simulink model "Model_6DOF_B3"  (R2020b)
settings: Solver=FixedStepAuto  StartTime=0.0  StopTime=120  FixedStep=0.05  RelTol=1e-3
values from neighbouring files (symbols this model uses):
  Ba_0 = [0 0 0 0 0 0]    [ctrl_mode_param.m]
  Bb = 4418825.3321    [load_data.m]
  Bv_0 = [tgt_speed 0 0 0 0 0]    [ctrl_mode_param.m]
  Bx_0 = [0 0 tgt_depth 0 0 0]    [ctrl_mode_param.m]
  Ixx = 5.23e7    (= 52300000)    [load_data.m]
  Ixy = 0    [load_data.m]
  Ixz = 0    [load_data.m]
  Iyy = 1.375e9    (= 1375000000)    [load_data.m]
  Iyz = 0    [load_data.m]
  Izz = 1.367e9    (= 1367000000)    [load_data.m]
  Mb = 4418825.3321    [load_data.m]
  Xb = 0    [load_data.m]
  Xg = 0    [load_data.m]
  Yb = 0    [load_data.m]
  Yg = 0    [load_data.m]
  Zb = 0.4406    [load_data.m]
  Zg = 0    [load_data.m]
undefined symbols (not defined in the file or in its folder): dA_BP1, dA_BP2, dA_Hull, dA_PH, dA_Sail, dA_SProot, dA_X1a, dA_X1b, dA_X2a, dA_X2b, dA_X3a, dA_X3b, dA_X4a, dA_X4b, its, n_BP1, n_BP2, n_Hull, n_PH, n_Sail, n_SProot, n_X1a, n_X1b, n_X2a, n_X2b, n_X3a, n_X3b, n_X4a, n_X4b, nt_BP1, nt_BP2, nt_Hull, nt_PH, nt_Sail, nt_SProot, nt_X1a, nt_X1b, nt_X2a, nt_X2b, nt_X3a, nt_X3b, nt_X4a, nt_X4b, Usp, vt1_BP1, vt1_BP2, vt1_Hull, vt1_PH, vt1_Sail, vt1_SProot, vt1_X1a, vt1_X1b, vt1_X2a, vt1_X2b, vt1_X3a, vt1_X3b, vt1_X4a, vt1_X4b, vt2_BP1, vt2_BP2 ... (+27)
libraries: simulink x5
(part 3 of 15)

== system Model_6DOF_B3/HDM 6DOF V1/Z 6d org ==
  Bx : Inport
  Bv : Inport  Port=2
  Ba : Inport  Port=3
  Alpha : Inport  Port=4
  Umag : Inport  Port=5
  dX : Inport  Port=6
  UeX : Inport  Port=7
  dLCG : Inport  Port=8
  dmass : Inport  Port=9
  Zvm : Inport  Port=10
  Fz : MATLAB Function  TreatAsAtomicUnit=on
  Product1 : Product
  Product3 : Product
  Saturation1 : Saturate  UpperLimit=0.04  LowerLimit=-0.04
  Saturation2 : Saturate  UpperLimit=0.0015  LowerLimit=-0.0015
  Saturation3 : Saturate  UpperLimit=0.02  LowerLimit=-0.02
  Selector1 : Selector  InputPortWidth=6  IndexOptions=Index vector (dialog)  Indices=3  OutputSizes=1
  Selector2 : Selector  InputPortWidth=6  IndexOptions=Index vector (dialog)  Indices=5  OutputSizes=1
  Selector3 : Selector  InputPortWidth=6  IndexOptions=Index vector (dialog)  Indices=3  OutputSizes=1
  Selector4 : Selector  InputPortWidth=6  IndexOptions=Index vector (dialog)  Indices=3  OutputSizes=1
  Selector7 : Selector  InputPortWidth=6  IndexOptions=Index vector (dialog)  Indices=1  OutputSizes=1
  To Workspace : ToWorkspace  VariableName=Zapp  SaveFormat=Timeseries  SampleTime=-1
  To Workspace1 : ToWorkspace  VariableName=Ztotal  SaveFormat=Timeseries  SampleTime=-1
  To Workspace2 : ToWorkspace  VariableName=Zstat  SaveFormat=Timeseries  SampleTime=-1
  To Workspace3 : ToWorkspace  VariableName=Zprop  SaveFormat=Timeseries  SampleTime=-1
  To Workspace4 : ToWorkspace  VariableName=Zhull  SaveFormat=Timeseries  SampleTime=-1
  Z'dwdt : MATLAB Function  TreatAsAtomicUnit=on
  Z'uq Prop : Lookup_n-D  BreakpointsForDimension1=|  BreakpointsForDimension2=[-7.71666 -5.14444 -3.086664 -1.543332]  Table=|  InternalRulePriority=Speed  RndMeth=Simplest  InputSameDT=on
      BreakpointsForDimension1=|
      | [-2.0E-01
      | -1.5E-01
      | -1.0E-01
      | -5.0E-02
      | 0.0E+00
      | 5.0E-02
      | 1.0E-01
      | 1.5E-01
      | 2.0E-01
      | ]
      Table=|
      | reshape([1.3913E-04
      | 1.0452E-04
      | 6.9900E-05
      | 3.5283E-05
      | 6.6700E-07
      | -3.3949E-05
      | -6.8566E-05
      | -1.0318E-04
      | -1.3780E-04
      | 2.8914E-04
      | 2.1702E-04
      | 1.4490E-04
      | 7.2785E-05
      | 6.6700E-07
      | -7.1451E-05
      | -1.4357E-04
      | -2.1569E-04
      | -2.8780E-04
      | 1.1606E-04
      | 8.7208E-05
      | 5.8361E-05
      | 2.9514E-05
      | 6.6700E-07
      | -2.8180E-05
      | -5.7027E-05
      | -8.5874E-05
      | -1.1472E-04
      | 1.1606E-04
      | 8.7208E-05
      | 5.8361E-05
      | 2.9514E-05
      | 6.6700E-07
      | -2.8180E-05
      | -5.7027E-05
      | -8.5874E-05
      | -1.1472E-04],[9,4])
      settings: InputPortMap=u0,u1
  Z'uvw : Lookup_n-D  NumberOfTableDimensions=3  BreakpointsForDimension1=|  BreakpointsForDimension2=|  BreakpointsForDimension3=|  Table=|  InternalRulePriority=Speed  RndMeth=Simplest  InputSameDT=on
      BreakpointsForDimension1=|
      | [-24
      | -16
      | -8
      | 0
      | 8
      | 16
      | 24]
      BreakpointsForDimension2=|
      | [-5.1444E+00
      | -3.0866E+00
      | -1.5433E+00
      | ]
      Table=|
      | reshape([-7.6517E-03
      | -4.8509E-03
      | -2.1091E-03
      | 3.8840E-04
      | 2.9798E-03
      | 6.0809E-03
      | 8.2821E-03
      | -7.5270E-03
      | -4.7702E-03
      | -1.9652E-03
      | 3.8840E-04
      | 2.9512E-03
      | 6.0573E-03
      | 8.1333E-03
      | -7.5193E-03
      | -4.5800E-03
      | -1.6681E-03
      | 3.8840E-04
      | 2.7791E-03
      | 5.8231E-03
      | 8.3050E-03
      | -6.2244E-03
      | -3.6100E-03
      | -9.9571E-04
      | 1.6186E-03
      | 4.2329E-03
      | 6.8473E-03
      | 9.4616E-03
      | -5.2515E-03
      | -2.9614E-03
      | -6.7142E-04
      | 1.6186E-03
      | 3.9086E-03
      | 6.1987E-03
      | 8.4887E-03
      | -4.1283E-03
      | -2.2126E-03
      | -2.9701E-04
      | 1.6186E-03
      | 3.5342E-03
      | 5.4499E-03
      | 7.3655E-03
      | -6.1999E-03
      | -3.5260E-03
      | -8.5205E-04
      | 1.8219E-03
      | 4.4958E-03
      | 7.1698E-03
      | 9.8437E-03
      | -4.9811E-03
      | -2.7134E-03
      | -4.4577E-04
      | 1.8219E-03
      | 4.0896E-03
      | 6.3572E-03
      | 8.6249E-03
      | -5.2821E-03
      | -2.9141E-03
      | -5.4610E-04
      | 1.8219E-03
      | 4.1899E-03
      | 6.5579E-03
      | 8.9259E-03
      | -6.1195E-03
      | -3.4239E-03
      | -7.2823E-04
      | 1.9674E-03
      | 4.6630E-03
      | 7.3587E-03
      | 1.0054E-02
      | -4.7022E-03
      | -2.4512E-03
      | -2.0024E-04
      | 1.9674E-03
      | 4.2184E-03
      | 6.4693E-03
      | 8.7203E-03
      | -3.4515E-03
      | -1.6452E-03
      | 1.6111E-04
      | 1.9674E-03
      | 3.7737E-03
      | 5.5800E-03
      | 7.3863E-03],[7,3,4])
      BreakpointsForDimension3=|
      | [-35.0624 -18.3724 -15.3724 -13.8724
      | ]
      settings: InputPortMap=u0,u1,u2
  ZdXi : Subsystem
  Zqq : Lookup_n-D  NumberOfTableDimensions=1  BreakpointsForDimension1=|  Table=|  InternalRulePriority=Speed  RndMeth=Simplest  InputSameDT=on
      BreakpointsForDimension1=|
      | [-0.02
      | -0.015
      | -0.012958963
      | -0.009719222
      | -0.006479482
      | -0.003239741
      | -0.00161987
      | -0.000647948
      | 0.000647948
      | 0.00161987
      | 0.003239741
      | 0.006479482
      | 0.009719222
      | 0.012958963
      | 0.015
      | 0.02
      | ]
      Table=|
      | [3.6478E-03
      | 3.8686E-03
      | 3.4313E-03
      | 4.0790E-03
      | 3.9500E-03
      | 3.6018E-03
      | 3.6796E-03
      | 3.5502E-03
      | 3.4310E-03
      | 3.4872E-03
      | 4.2239E-03
      | 4.0934E-03
      | 3.0314E-03
      | 2.5726E-03
      | 2.9188E-03
      | 2.7740E-03
      | ]
  Zuq : Lookup_n-D  NumberOfTableDimensions=1  BreakpointsForDimension1=|  Table=|  InternalRulePriority=Speed  RndMeth=Simplest  InputSameDT=on
      BreakpointsForDimension1=|
      | [-0.04
      | -0.03
      | -0.02
      | -0.01
      | -0.005
      | -0.002
      | 0.002
      | 0.005
      | 0.01
      | 0.02
      | 0.03
      | 0.04
      | ]
      Table=|
      | [-9.8908E-03
      | -9.0784E-03
      | -8.9566E-03
      | -1.0733E-02
      | -1.4141E-02
      | -2.4189E-02
      | -6.5605E-03
      | -7.1594E-03
      | -7.6366E-03
      | -7.9008E-03
      | -6.1794E-03
      | -6.1029E-03
      | ]
  Zwq : Lookup_n-D  NumberOfTableDimensions=1  BreakpointsForDimension1=|  Table=|  InternalRulePriority=Speed  RndMeth=Simplest  InputSameDT=on
      BreakpointsForDimension1=|
      | [-0.0015
      | -0.0012
      | -0.0009
      | -0.0006
      | -0.0003
      | -0.0001
      | 0.0001
      | 0.0003
      | 0.0006
      | 0.0009
      | 0.0012
      | 0.0015]
      Table=|
      | [-2.9784E-01
      | -2.6725E-01
      | -2.3292E-01
      | -2.0077E-01
      | -1.1489E-01
      | -7.6673E-03
      | -7.5516E-03
      | -1.1617E-01
      | -2.0077E-01
      | -2.9128E-01
      | -3.5974E-01
      | -4.7839E-01]
  Z : Outport
  wires:
  Selector7/1 -> Z'uvw/2, Z'uq Prop/2, Product3/2
  Selector2/1 -> Product1/1, Saturation3/1, Product3/1
  Alpha/1 -> Z'uvw/1
  Bv/1 -> Selector7/1, Selector3/1, Selector2/1, Fz/2(Bv)
  Umag/1 -> Fz/10(Umag)
  Bx/1 -> Selector4/1, Fz/1(Bx)
  Product3/1 -> Saturation1/1, Z'uq Prop/1
  UeX/1 -> Fz/11(UeX)
  Selector3/1 -> Product1/2
  Product1/1 -> Saturation2/1
  Ba/1 -> Selector1/1, Fz/3(Ba)
  dLCG/1 -> Fz/12(dLCG)
  dmass/1 -> Fz/13(dmass)
  Selector1/1 -> Z'dwdt/1(a3)
  dX/1 -> ZdXi/1(dX)
  Saturation1/1 -> Zuq/1
  Saturation2/1 -> Zwq/1
  Saturation3/1 -> Zqq/1
  Zwq/1 -> Fz/6(Zwq)
  Fz/1(FZ) -> To Workspace1/1, Z/1
  Zqq/1 -> Fz/4(Zqq)
  Zuq/1 -> Fz/5(Zuq)
  ZdXi/1(ZdX) -> Fz/14(ZdXi)
  Z'dwdt/1(Zdwdt) -> Fz/9(Zdwdt)
  Z'uq Prop/1 -> Fz/8(CZProp)
  Zvm/1 -> Fz/15(Zvm)
  Selector4/1 -> ZdXi/2(z), Z'uvw/3
  Z'uvw/1 -> Fz/7(Zuvw)
  Fz/2(FZApp) -> To Workspace/1
  Fz/5(FZhull) -> To Workspace4/1
  Fz/4(FZprop) -> To Workspace3/1
  Fz/3(FZstat) -> To Workspace2/1

== system Model_6DOF_B3/HDM B1/Effective Veloicity Calclation ==
  Bv : Inport
  uwsXi : Inport  Port=2
  uwsCG : Inport  Port=3
  Add{,1..4} (5 alike) : Sum
  Demux : Demux  Outputs=5
  Demux1 : Demux  Outputs=3
  Demux2 : Demux  Outputs=5
  Gain : Gain
  Gain1 : Gain
  Gain2 : Gain
  MATLAB Function : MATLAB Function  TreatAsAtomicUnit=on
  MATLAB Function1 : MATLAB Function  TreatAsAtomicUnit=on
  MATLAB Function2 : MATLAB Function  TreatAsAtomicUnit=on
  X_SP1 : Constant  Value=[31.924; 3.861; -3.861;]
  X_SP2 : Constant  Value=[31.924; 3.861; 3.861;]
  X_SP3 : Constant  Value=[31.924; -3.861; 3.861;]
  X_SP4 : Constant  Value=[31.924; -3.861; -3.861;]
  X_XB : Constant  Value=[-10.465; 0; 9.732;]
  aX : Scope  NumInputPorts=5
  n1 : Constant  Value=[0; 1/sqrt(2); -1/sqrt(2);]
  n2 : Constant  Value=[0; 1/sqrt(2); 1/sqrt(2);]
  n3 : Constant  Value=[0; -1/sqrt(2); 1/sqrt(2);]
  n4 : Constant  Value=[0; -1/sqrt(2); -1/sqrt(2);]
  n5 : Constant  Value=[0; 1; 0;]
  nh : Constant  Value=[-1; 0; 0;]
  urXi : Scope  NumInputPorts=5
  Alpha : Outport
  Beta : Outport  Port=2
  Umag : Outport  Port=3
  aXi : Outport  Port=4
  UeX : Outport  Port=5
  wires:
  uwsXi/1 -> Gain2/1
  Gain2/1 -> Demux/1
  Gain1/1 -> aXi/1
  Gain/1 -> Alpha/1
  uwsCG/1 -> Demux1/1
  Demux2/5 -> aX/5
  Demux2/4 -> aX/4
  Demux2/3 -> aX/3
  Demux2/2 -> aX/2
  Demux2/1 -> aX/1
  Demux1/3 -> MATLAB Function2/4(wCG)
  Demux1/2 -> MATLAB Function2/3(vCG)
  Demux1/1 -> MATLAB Function2/2(uCG)
  MATLAB Function/2(UeX) -> UeX/1
  MATLAB Function2/3(Umag) -> Umag/1
  MATLAB Function2/2(beta) -> Beta/1
  MATLAB Function2/1(alpha) -> Gain/1
  MATLAB Function1/2(urX2) -> urXi/2, Add1/1
  MATLAB Function1/3(urX3) -> urXi/3, Add2/1
  MATLAB Function1/4(urX4) -> urXi/4, Add3/1
  MATLAB Function1/5(urXB) -> urXi/5, Add4/1
  Demux/5 -> Add4/2
  Demux/4 -> Add3/2
  Demux/3 -> Add2/2
  Demux/2 -> Add1/2
  Add4/1 -> MATLAB Function/11(urXB)
  Add3/1 -> MATLAB Function/10(urX4)
  Add2/1 -> MATLAB Function/9(urX3)
  Add1/1 -> MATLAB Function/8(urX2)
  Add/1 -> MATLAB Function/7(urX1)
  Demux/1 -> Add/2
  MATLAB Function/1(aX) -> Demux2/1, Gain1/1
  MATLAB Function1/1(urX1) -> urXi/1, Add/1
  n5/1 -> MATLAB Function/6(nB)
  X_SP1/1 -> MATLAB Function1/1(rX1)
  X_SP4/1 -> MATLAB Function1/4(rX4)
  X_SP3/1 -> MATLAB Function1/3(rX3)
  X_SP2/1 -> MATLAB Function1/2(rX2)
  X_XB/1 -> MATLAB Function1/5(rXB)
  n4/1 -> MATLAB Function/5(n4)
  n3/1 -> MATLAB Function/4(n3)
  n2/1 -> MATLAB Function/3(n2)
  n1/1 -> MATLAB Function/2(n1)
  nh/1 -> MATLAB Function/1(nh)
  Bv/1 -> MATLAB Function2/1(Bv), MATLAB Function1/6(U_ship)

== system Model_6DOF_B3/HDM B1/Effective dX Calculation ==
  dX CTRL : Inport
  aXi : Inport  Port=2
  Add{,1..4} (5 alike) : Sum
  Demux : Demux  Outputs=5
  Demux1 : Demux  Outputs=5
  Mux6 : Mux  Inputs=5
  dXeff : Outport
  wires:
  Mux6/1 -> dXeff/1
  Demux1/5 -> Add4/2
  Demux1/4 -> Add3/2
  Demux1/3 -> Add2/2
  Demux1/2 -> Add1/2
  Demux1/1 -> Add/2
  Demux/5 -> Add4/1
  Demux/4 -> Add3/1
  Demux/3 -> Add2/1
  Demux/2 -> Add1/1
  Demux/1 -> Add/1
  Add4/1 -> Mux6/5
  Add3/1 -> Mux6/4
  Add2/1 -> Mux6/3
  Add1/1 -> Mux6/2
  Add/1 -> Mux6/1
  aXi/1 -> Demux1/1
  dX CTRL/1 -> Demux/1

== system Model_6DOF_B3/HDM B1/K ==
  Bx : Inport
  Bv : Inport  Port=2
  Ba : Inport  Port=3
  Beta : Inport  Port=4
  Umag : Inport  Port=5
  dX : Inport  Port=6
  UeX : Inport  Port=7
  dLCG : Inport  Port=8
  dmass : Inport  Port=9
  Kvm : Inport  Port=10
  BFM : Inport  Port=11
  Abs : Abs
  Abs1 : Abs
  Abs2 : Abs
  Gain : Gain
  Gain1 : Gain
  Gain2 : Gain
  K'p|p| : Lookup_n-D  NumberOfTableDimensions=1  BreakpointsForDimension1=|  Table=|  InternalRulePriority=Speed  RndMeth=Simplest  InputSameDT=on
      BreakpointsForDimension1=|
      | [-0.0015
      | -0.0012
      | -0.0009
      | -0.0006
      | -0.0003
      | -0.0001
      | 0.0001
      | 0.0003
      | 0.0006
      | 0.0009
      | 0.0012
      | 0.0015]
      Table=|
      | [-1.3011E-02
      | -1.6962E-02
      | -2.0682E-02
      | -3.1419E-02
      | -6.4407E-02
      | -1.9322E-01
      | 1.9322E-01
      | 6.4378E-02
      | 3.1944E-02
      | 2.1072E-02
      | 1.6415E-02
      | 1.3407E-02]
  K'up : Lookup_n-D  NumberOfTableDimensions=1  BreakpointsForDimension1=|  Table=|  InternalRulePriority=Speed  RndMeth=Simplest  InputSameDT=on
      BreakpointsForDimension1=|
      | [0.03999989
      | 0.079999993
      | 0.11999963
      | 0.15999956]
      Table=|
      | [-4.0344E-04
      | -8.1402E-04
      | -1.2116E-03
      | -1.6125E-03]
  K'ur : Lookup_n-D  NumberOfTableDimensions=1  BreakpointsForDimension1=|  Table=|  InternalRulePriority=Speed  RndMeth=Simplest  InputSameDT=on
      BreakpointsForDimension1=|
      | [-0.0015
      | -0.0012
      | -0.0009
      | -0.0006
      | -0.0003
      | -0.0001
      | 0.0001
      | 0.0003
      | 0.0006
      | 0.0009
      | 0.0012
      | 0.0015]
      Table=|
      | [-1.3011E-02
      | -1.6962E-02
      | -2.0682E-02
      | -3.1419E-02
      | -6.4407E-02
      | -1.9322E-01
      | 1.9322E-01
      | 6.4378E-02
      | 3.1944E-02
      | 2.1072E-02
      | 1.6415E-02
      | 1.3407E-02]
  K'uvw : Lookup_n-D  NumberOfTableDimensions=3  BreakpointsForDimension1=|  BreakpointsForDimension2=|  BreakpointsForDimension3=|  Table=|  InternalRulePriority=Speed  RndMeth=Simplest  InputSameDT=on
      BreakpointsForDimension1=|
      | [0
      | 4
      | 8
      | 12]
      BreakpointsForDimension2=|
      | [-5.1444E+00
      | -3.0866E+00
      | -1.5433E+00
      | ]
      Table=|
      | reshape([0.0000000E+00
      | 1.5570290E-04
      | 3.7677829E-04
      | 6.0025374E-04
      | 0.0000000E+00
      | 1.5575678E-04
      | 3.8557685E-04
      | 6.0103850E-04
      | 0.0000000E+00
      | 1.7511088E-04
      | 3.8376789E-04
      | 6.0108480E-04
      | 0.0000000E+00
      | 1.9071552E-04
      | 4.0986649E-04
      | 6.4012030E-04
      | 0.0000000E+00
      | 1.8940622E-04
      | 4.0946931E-04
      | 6.3613461E-04
      | 0.0000000E+00
      | 1.8621071E-04
      | 4.0619654E-04
      | 7.0286379E-04
      | 0.0000000E+00
      | 2.0712189E-04
      | 4.4751988E-04
      | 7.0514631E-04
      | 0.0000000E+00
      | 1.9895751E-04
      | 4.3099356E-04
      | 6.6994571E-04
      | 0.0000000E+00
      | 1.9568554E-04
      | 4.2679977E-04
      | 6.6445067E-04
      | 0.0000000E+00
      | 2.4359563E-04
      | 5.3740096E-04
      | 8.5879902E-04
      | 0.0000000E+00
      | 2.0890025E-04
      | 4.5502130E-04
      | 7.1388224E-04
      | 0.0000000E+00
      | 2.0575072E-04
      | 4.5505766E-04
      | 7.0285206E-04],[4,3,4])
      BreakpointsForDimension3=|
      | [-35.0624 -18.3724 -15.3724 -13.8724
      | ]
      settings: InputPortMap=u0,u1,u2
  KdXi : Subsystem
  Mux : Mux  Inputs=7
  Mx : MATLAB Function  TreatAsAtomicUnit=on
  Product{,1..2,4..5} (5 alike) : Product
  Saturation4 : Saturate  UpperLimit=-13.8724  LowerLimit=-35.0624
  Scope : Scope
  Selector1 : Selector  InputPortWidth=6  IndexOptions=Index vector (dialog)  Indices=4  OutputSizes=1
  Selector10 : Selector  InputPortWidth=6  IndexOptions=Index vector (dialog)  Indices=1  OutputSizes=1
  Selector2 : Selector  InputPortWidth=6  IndexOptions=Index vector (dialog)  Indices=3  OutputSizes=1
  Selector4 : Selector  InputPortWidth=6  IndexOptions=Index vector (dialog)  Indices=4  OutputSizes=1
  Selector8 : Selector  InputPortWidth=6  IndexOptions=Index vector (dialog)  Indices=2  OutputSizes=1
  Sign : Signum
  Sign1 : Signum
  To Workspace : ToWorkspace  VariableName=K_total  SaveFormat=Timeseries  SampleTime=-1
  To Workspace1 : ToWorkspace  VariableName=AppK_All  SaveFormat=Timeseries  SampleTime=-1
  To Workspace2 : ToWorkspace  VariableName=KHullVM  SaveFormat=Timeseries  SampleTime=-1
  To Workspace3 : ToWorkspace  VariableName=Kvm  SaveFormat=Timeseries  SampleTime=-1
  To Workspace8 : ToWorkspace  VariableName=Benchmark_K  SaveFormat=Timeseries  SampleTime=-1
  K : Outport
  wires:
  Kvm/1 -> Mux/5, To Workspace3/1, Mx/13(Kvm)
  Mx/8(KHullVM) -> To Workspace2/1
  Saturation4/1 -> K'uvw/3, KdXi/3(z)  "z"
  [K_Stat] -> Mux/7
  Gain2/1 -> Mx/5(CKur)
  Gain1/1 -> Mx/4(CKup)
  Gain/1 -> Product2/1
  Mx/7(KStat) -> [K_Stat]
  Mx/1(K) -> K/1, To Workspace/1, Mux/6, Scope/1
  Selector1/1 -> Mx/14(BFK)
  BFM/1 -> Selector1/1
  Mx/6(KAppAll) -> To Workspace1/1
  Mx/5(Kpp) -> Mux/4
  Mx/4(Kh_total) -> Mux/3
  Mx/3(K_hull) -> Mux/2
  Mx/2(KApp) -> Mux/1
  Mux/1 -> To Workspace8/1
  Sign1/1 -> Gain/1
  Abs2/1 -> K'uvw/1
  Product2/1 -> Mx/7(CKuvw)
  Product/1 -> Gain1/1
  Sign/1 -> Product/1
  Abs1/1 -> K'up/1
  Product1/1 -> Abs1/1, Sign/1
  K'uvw/1 -> Product2/2
  Selector2/1 -> Saturation4/1
  KdXi/1(KdXi) -> Mx/12(CNdXi)
  K'ur/1 -> Mx/6(CKpp)
  Selector4/1 -> Product4/2, Abs/1, Product5/2, Product1/2
  Product5/1 -> K'p|p|/1
  Abs/1 -> Product5/1
  Selector8/1 -> Product4/1
  Product4/1 -> K'ur/1
  K'p|p|/1 -> Gain2/1
  K'up/1 -> Product/2
  dX/1 -> KdXi/1(dX)
  dmass/1 -> Mx/11(dmass)
  dLCG/1 -> Mx/10(dLCG)
  Umag/1 -> Mx/8(Umag)
  Beta/1 -> Abs2/1, Sign1/1
  UeX/1 -> Mx/9(UeX)
  Ba/1 -> Mx/3(Ba)
  Selector10/1 -> Product1/1, K'uvw/2
  Bx/1 -> Selector2/1, Mx/1(Bx)
  Bv/1 -> Mx/2(Bv), Selector8/1, Selector4/1, Selector10/1

== system Model_6DOF_B3/HDM B1/M ==
  Bx : Inport
  Bv : Inport  Port=2
  Ba : Inport  Port=3
  Alpha : Inport  Port=4
  Umag : Inport  Port=5
  dX : Inport  Port=6
  UeSP : Inport  Port=7
  dLCG : Inport  Port=8
  dmass : Inport  Port=9
  Mvm : Inport  Port=10
  BFM : Inport  Port=11
  Abs : Abs
  Gain : Gain  Gain=1.1
  Gain1 : Gain  Gain=1.3
  M'prop : Lookup_n-D  NumberOfTableDimensions=1  BreakpointsForDimension1=[-7.7166666 -5.1444444 -3.08666664]  Table=[-0.00022 -0.0002 -0.00015]  InternalRulePriority=Speed  RndMeth=Simplest  InputSameDT=on
  M'uvw : Lookup_n-D  NumberOfTableDimensions=3  BreakpointsForDimension1=|  BreakpointsForDimension2=|  BreakpointsForDimension3=|  Table=|  InternalRulePriority=Speed  RndMeth=Simplest  InputSameDT=on
      BreakpointsForDimension1=|
      | [-12
      | -8
      | -4
      | 0
      | 4
      | 8
      | 12]
      BreakpointsForDimension2=|
      | [-5.1444E+00
      | -3.0866E+00
      | -1.5433E+00
      | ]
      Table=|
      | reshape([-2.40251E-03
      | -1.59538E-03
      | -8.21748E-04
      | -3.60182E-06
      | 8.13350E-04
      | 1.50586E-03
      | 2.39707E-03
      | -2.43392E-03
      | -1.61509E-03
      | -8.50748E-04
      | -3.60182E-06
      | 8.24271E-04
      | 1.51842E-03
      | 2.43805E-03
      | -2.45014E-03
      | -1.65711E-03
      | -9.11210E-04
      | -3.60182E-06
      | 8.61300E-04
      | 1.57459E-03
      | 2.42777E-03
      | -2.54380E-03
      | -1.68842E-03
      | -8.33041E-04
      | 2.23377E-05
      | 8.77717E-04
      | 1.73310E-03
      | 2.58847E-03
      | -2.63734E-03
      | -1.75078E-03
      | -8.64221E-04
      | 2.23377E-05
      | 9.08896E-04
      | 1.79546E-03
      | 2.68201E-03
      | -2.83738E-03
      | -1.88414E-03
      | -9.30902E-04
      | 2.23377E-05
      | 9.75577E-04
      | 1.92882E-03
      | 2.88206E-03
      | -2.63786E-03
      | -1.74504E-03
      | -8.52211E-04
      | 4.06140E-05
      | 9.33439E-04
      | 1.82626E-03
      | 2.71909E-03
      | -2.63728E-03
      | -1.74465E-03
      | -8.52017E-04
      | 4.06140E-05
      | 9.33245E-04
      | 1.82588E-03
      | 2.71851E-03
      | -2.86138E-03
      | -1.89405E-03
      | -9.26716E-04
      | 4.06140E-05
      | 1.00794E-03
      | 1.97527E-03
      | 2.94260E-03
      | -0.002723494
      | -0.001792522
      | -0.000861549
      | 6.9423E-05
      | 0.001000396
      | 0.001931368
      | 0.002862341
      | -0.002736476
      | -0.001798489
      | -0.000860502
      | 6.9423E-05
      | 0.001015473
      | 0.00195346
      | 0.002891447
      | -0.002765582
      | -0.00182058
      | -0.000875579
      | 6.9423E-05
      | 0.001014425
      | 0.001959426
      | 0.002904428],[7,3,4])
      BreakpointsForDimension3=|
      | [-35.0624 -18.3724 -15.3724 -13.8724
      | ]
      settings: InputPortMap=u0,u1,u2
  Mdxi : Subsystem
  Mqq2 : Lookup_n-D  NumberOfTableDimensions=1  BreakpointsForDimension1=|  Table=|  InternalRulePriority=Speed  RndMeth=Simplest  InputSameDT=on
      BreakpointsForDimension1=|
      | [-0.02
      | -0.015
      | -0.012958963
      | -0.009719222
      | -0.006479482
      | -0.003239741
      | -0.00161987
      | -0.000647948
      | 0.000647948
      | 0.00161987
      | 0.003239741
      | 0.006479482
      | 0.009719222
      | 0.012958963
      | 0.015
      | 0.02
      | ]
      Table=|
      | [-2.2571E-03
      | -2.3029E-03
      | -2.0965E-03
      | -2.0229E-03
      | -2.1546E-03
      | -1.4789E-03
      | -1.5664E-03
      | -1.4544E-03
      | -1.4705E-03
      | -1.4942E-03
      | -1.8790E-03
      | -1.8821E-03
      | -2.1009E-03
      | -2.0521E-03
      | -2.1685E-03
      | -2.0822E-03
      | ]
  Muq : Lookup_n-D  Commented=on  BreakpointsForDimension1=|  BreakpointsForDimension2=|  Table=|  InternalRulePriority=Speed  RndMeth=Simplest  InputSameDT=on
      BreakpointsForDimension1=|
      | [-2.00E-01
      | -1.50E-01
      | -1.00E-01
      | -5.00E-02
      | 0.00E+00
      | 5.00E-02
      | 1.00E-01
      | 1.50E-01
      | 2.00E-01
      | ]
      Table=|
      | reshape([-3.95902E-04
      | -2.96922E-04
      | -1.97952E-04
      | -9.89720E-05
      | 0.00000E+00
      | 9.89750E-05
      | 1.97948E-04
      | 2.96928E-04
      | 3.95898E-04
      | -4.94864E-04
      | -3.71144E-04
      | -2.47434E-04
      | -1.23714E-04
      | 0.00000E+00
      | 1.23715E-04
      | 2.47426E-04
      | 3.71146E-04
      | 4.94856E-04
      | -5.69298E-04
      | -4.26978E-04
      | -2.84648E-04
      | -1.42328E-04
      | 0.00000E+00
      | 1.42322E-04
      | 2.84652E-04
      | 4.26972E-04
      | 5.69302E-04
      | -5.60922E-04
      | -4.20692E-04
      | -2.80462E-04
      | -1.40232E-04
      | 0.00000E+00
      | 1.40228E-04
      | 2.80458E-04
      | 4.20688E-04
      | 5.60918E-04],[9,4])
      BreakpointsForDimension2=|
      | [-7.7166 -5.1444 -3.08664 -1.54332
      | ]
      settings: InputPortMap=u0,u1
  Mux1 : Mux  Inputs=7
  Mwq : Lookup_n-D  NumberOfTableDimensions=1  BreakpointsForDimension1=|  Table=|  InternalRulePriority=Speed  RndMeth=Simplest  InputSameDT=on
      BreakpointsForDimension1=|
      | [-0.0015
      | -0.0012
      | -0.0009
      | -0.0006
      | -0.0003
      | -0.0001
      | 0.0001
      | 0.0003
      | 0.0006
      | 0.0009
      | 0.0012
      | 0.0015]
      Table=|
      | [-1.3011E-02
      | -1.6962E-02
      | -2.0682E-02
      | -3.1419E-02
      | -6.4407E-02
      | -1.9322E-01
      | 1.9322E-01
      | 6.4378E-02
      | 3.1944E-02
      | 2.1072E-02
      | 1.6415E-02
      | 1.3407E-02]
  My : MATLAB Function  TreatAsAtomicUnit=on
  Product5 : Product
  Saturation2 : Saturate  UpperLimit=0.0015  LowerLimit=-0.0015
  Saturation3 : Saturate  UpperLimit=0.02  LowerLimit=-0.02
  Saturation4 : Saturate  UpperLimit=-13.8724  LowerLimit=-35.0624
  Selector1 : Selector  InputPortWidth=6  IndexOptions=Index vector (dialog)  Indices=5  OutputSizes=1
  Selector10 : Selector  InputPortWidth=6  IndexOptions=Index vector (dialog)  Indices=1  OutputSizes=1
  Selector2 : Selector  InputPortWidth=6  IndexOptions=Index vector (dialog)  Indices=3  OutputSizes=1
  Selector4 : Selector  InputPortWidth=6  IndexOptions=Index vector (dialog)  Indices=5  OutputSizes=1
  Selector8 : Selector  InputPortWidth=6  IndexOptions=Index vector (dialog)  Indices=3  OutputSizes=1
  To Workspace1 : ToWorkspace  VariableName=AppM_All  SaveFormat=Timeseries  SampleTime=-1
  To Workspace3 : ToWorkspace  VariableName=Benchmark_M  SaveFormat=Timeseries  SampleTime=-1
  M : Outport
  wires:
  [M_stat] -> Mux1/7
  Gain1/1 -> My/12(MdXi)
  My/4(Mprop) -> [M_Prop]
  My/6(MY_hyd) -> [M_Hyd]
  My/5(M_hull) -> [M_Hull]
  My/2(MYApp) -> [M_App]
  [M_Total] -> Mux1/6
  [M_Hull] -> Mux1/2
  Mux1/1 -> To Workspace3/1
  [M_Hyd] -> Mux1/3
  [M_App] -> Mux1/1
  [M_Prop] -> Mux1/4
  [Mvm] -> Mux1/5
  Selector1/1 -> My/14(BFM)
  BFM/1 -> Selector1/1
  My/7(MYApp_All) -> To Workspace1/1
  Gain/1 -> My/7(Muvw)
  Saturation4/1 -> M'uvw/3, Mdxi/2(z)  "z"
  My/3(MYStat) -> [M_stat]
  Bv/1 -> My/2(Bv), Selector4/1, Selector8/1, Selector10/1
  Bx/1 -> Selector2/1, My/1(Bx)
  Selector10/1 -> M'prop/1, M'uvw/2  "speed"
  Ba/1 -> My/3(Ba)
  M'prop/1 -> My/6("Mprop ")
  UeSP/1 -> My/9(UeSP)
  Selector4/1 -> Saturation3/1, Abs/1
  Alpha/1 -> M'uvw/1  "AOA"
  Umag/1 -> My/8(Umag)
  dLCG/1 -> My/10(dLCG)
  dmass/1 -> My/11(dmass)
  dX/1 -> Mdxi/1(dX)
  Mqq2/1 -> My/4(Mqq)
  Mwq/1 -> My/5(Mwq)
  Product5/1 -> Saturation2/1
  Selector8/1 -> Product5/2
  Abs/1 -> Product5/1
  Saturation2/1 -> Mwq/1
  Saturation3/1 -> Mqq2/1
  My/1(MY) -> [M_Total], M/1
  Mdxi/1(MdX) -> Gain1/1
  Mvm/1 -> [Mvm], My/13(Mvm)
  Selector2/1 -> Saturation4/1
  M'uvw/1 -> Gain/1

== system Model_6DOF_B3/HDM B1/M 6d org ==
  Bx : Inport
  Bv : Inport  Port=2
  Ba : Inport  Port=3
  Alpha : Inport  Port=4
  Umag : Inport  Port=5
  dX : Inport  Port=6
  UeX : Inport  Port=7
  dLCG : Inport  Port=8
  dmass : Inport  Port=9
  Mvm : Inport  Port=10
  M'prop : Lookup_n-D  NumberOfTableDimensions=1  BreakpointsForDimension1=[-7.7166666 -5.1444444 -3.08666664]  Table=[-0.00022 -0.0002 -0.00015]  InternalRulePriority=Speed  RndMeth=Simplest  InputSameDT=on
  M'uvw : Lookup_n-D  NumberOfTableDimensions=3  BreakpointsForDimension1=|  BreakpointsForDimension2=|  BreakpointsForDimension3=|  Table=|  InternalRulePriority=Speed  RndMeth=Simplest  InputSameDT=on
      BreakpointsForDimension1=|
      | [-12
      | -8
      | -4
      | 0
      | 4
      | 8
      | 12]
      BreakpointsForDimension2=|
      | [-5.1444E+00
      | -3.0866E+00
      | -1.5433E+00
      | ]
      Table=|
      | reshape([-2.40251E-03
      | -1.59538E-03
      | -8.21748E-04
      | -3.60182E-06
      | 8.13350E-04
      | 1.50586E-03
      | 2.39707E-03
      | -2.43392E-03
      | -1.61509E-03
      | -8.50748E-04
      | -3.60182E-06
      | 8.24271E-04
      | 1.51842E-03
      | 2.43805E-03
      | -2.45014E-03
      | -1.65711E-03
      | -9.11210E-04
      | -3.60182E-06
      | 8.61300E-04
      | 1.57459E-03
      | 2.42777E-03
      | -2.54380E-03
      | -1.68842E-03
      | -8.33041E-04
      | 2.23377E-05
      | 8.77717E-04
      | 1.73310E-03
      | 2.58847E-03
      | -2.63734E-03
      | -1.75078E-03
      | -8.64221E-04
      | 2.23377E-05
      | 9.08896E-04
      | 1.79546E-03
      | 2.68201E-03
      | -2.83738E-03
      | -1.88414E-03
      | -9.30902E-04
      | 2.23377E-05
      | 9.75577E-04
      | 1.92882E-03
      | 2.88206E-03
      | -2.63786E-03
      | -1.74504E-03
      | -8.52211E-04
      | 4.06140E-05
      | 9.33439E-04
      | 1.82626E-03
      | 2.71909E-03
      | -2.63728E-03
      | -1.74465E-03
      | -8.52017E-04
      | 4.06140E-05
      | 9.33245E-04
      | 1.82588E-03
      | 2.71851E-03
      | -2.86138E-03
      | -1.89405E-03
      | -9.26716E-04
      | 4.06140E-05
      | 1.00794E-03
      | 1.97527E-03
      | 2.94260E-03
      | -0.002723494
      | -0.001792522
      | -0.000861549
      | 6.9423E-05
      | 0.001000396
      | 0.001931368
      | 0.002862341
      | -0.002736476
      | -0.001798489
      | -0.000860502
      | 6.9423E-05
      | 0.001015473
      | 0.00195346
      | 0.002891447
      | -0.002765582
      | -0.00182058
      | -0.000875579
      | 6.9423E-05
      | 0.001014425
      | 0.001959426
      | 0.002904428],[7,3,4])
      BreakpointsForDimension3=|
      | [-35.0624 -18.3724 -15.3724 -13.8724
      | ]
      settings: InputPortMap=u0,u1,u2
  MATLAB Function2 : MATLAB Function  TreatAsAtomicUnit=on
  Mdxi : Subsystem
  Mqq2 : Lookup_n-D  NumberOfTableDimensions=1  BreakpointsForDimension1=|  Table=|  InternalRulePriority=Speed  RndMeth=Simplest  InputSameDT=on
      BreakpointsForDimension1=|
      | [-0.02
      | -0.015
      | -0.012958963
      | -0.009719222
      | -0.006479482
      | -0.003239741
      | -0.00161987
      | -0.000647948
      | 0.000647948
      | 0.00161987
      | 0.003239741
      | 0.006479482
      | 0.009719222
      | 0.012958963
      | 0.015
      | 0.02
      | ]
      Table=|
      | [-2.2571E-03
      | -2.3029E-03
      | -2.0965E-03
      | -2.0229E-03
      | -2.1546E-03
      | -1.4789E-03
      | -1.5664E-03
      | -1.4544E-03
      | -1.4705E-03
      | -1.4942E-03
      | -1.8790E-03
      | -1.8821E-03
      | -2.1009E-03
      | -2.0521E-03
      | -2.1685E-03
      | -2.0822E-03
      | ]
  Muq : Lookup_n-D  BreakpointsForDimension1=|  BreakpointsForDimension2=|  Table=|  InternalRulePriority=Speed  RndMeth=Simplest  InputSameDT=on
      BreakpointsForDimension1=|
      | [-2.00E-01
      | -1.50E-01
      | -1.00E-01
      | -5.00E-02
      | 0.00E+00
      | 5.00E-02
      | 1.00E-01
      | 1.50E-01
      | 2.00E-01
      | ]
      Table=|
      | reshape([-3.95902E-04
      | -2.96922E-04
      | -1.97952E-04
      | -9.89720E-05
      | 0.00000E+00
      | 9.89750E-05
      | 1.97948E-04
      | 2.96928E-04
      | 3.95898E-04
      | -4.94864E-04
      | -3.71144E-04
      | -2.47434E-04
      | -1.23714E-04
      | 0.00000E+00
      | 1.23715E-04
      | 2.47426E-04
      | 3.71146E-04
      | 4.94856E-04
      | -5.69298E-04
      | -4.26978E-04
      | -2.84648E-04
      | -1.42328E-04
      | 0.00000E+00
      | 1.42322E-04
      | 2.84652E-04
      | 4.26972E-04
      | 5.69302E-04
      | -5.60922E-04
      | -4.20692E-04
      | -2.80462E-04
      | -1.40232E-04
      | 0.00000E+00
      | 1.40228E-04
      | 2.80458E-04
      | 4.20688E-04
      | 5.60918E-04],[9,4])
      BreakpointsForDimension2=|
      | [-7.7166 -5.1444 -3.08664 -1.54332
      | ]
      settings: InputPortMap=u0,u1
  Mwq : Lookup_n-D  NumberOfTableDimensions=1  BreakpointsForDimension1=|  Table=|  InternalRulePriority=Speed  RndMeth=Simplest  InputSameDT=on
      BreakpointsForDimension1=|
      | [-0.0015
      | -0.0012
      | -0.0009
      | -0.0006
      | -0.0003
      | -0.0001
      | 0.0001
      | 0.0003
      | 0.0006
      | 0.0009
      | 0.0012
      | 0.0015]
      Table=|
      | [-1.3011E-02
      | -1.6962E-02
      | -2.0682E-02
      | -3.1419E-02
      | -6.4407E-02
      | -1.9322E-01
      | 1.9322E-01
      | 6.4378E-02
      | 3.1944E-02
      | 2.1072E-02
      | 1.6415E-02
      | 1.3407E-02]
  My : MATLAB Function  TreatAsAtomicUnit=on
  Product4 : Product
  Product5 : Product
  Saturation2 : Saturate  UpperLimit=0.0015  LowerLimit=-0.0015
  Saturation3 : Saturate  UpperLimit=0.02  LowerLimit=-0.02
  Selector10 : Selector  InputPortWidth=6  IndexOptions=Index vector (dialog)  Indices=1  OutputSizes=1
  Selector2 : Selector  InputPortWidth=6  IndexOptions=Index vector (dialog)  Indices=3  OutputSizes=1
  Selector4 : Selector  InputPortWidth=6  IndexOptions=Index vector (dialog)  Indices=5  OutputSizes=1
  Selector8 : Selector  InputPortWidth=6  IndexOptions=Index vector (dialog)  Indices=3  OutputSizes=1
  To Workspace : ToWorkspace  VariableName=MApp  SaveFormat=Timeseries  SampleTime=-1
  To Workspace1 : ToWorkspace  VariableName=MStat  SaveFormat=Timeseries  SampleTime=-1
  To Workspace2 : ToWorkspace  VariableName=MHull  SaveFormat=Timeseries  SampleTime=-1
  To Workspace3 : ToWorkspace  VariableName=Mprop  SaveFormat=Timeseries  SampleTime=-1
  To Workspace4 : ToWorkspace  VariableName=Mtotal  SaveFormat=Timeseries  SampleTime=-1
  M : Outport
  wires:
  My/4(MYhull) -> To Workspace2/1
  My/5(MYprop) -> To Workspace3/1
  My/3(MYStat) -> To Workspace1/1
  My/2(MYApp) -> To Workspace/1
  M'uvw/1 -> My/8(Muvw)
  Selector2/1 -> Mdxi/2(z), M'uvw/3
  Mvm/1 -> My/14(Mvm)
  Mdxi/1(MdX) -> My/13(MdXi)
  My/1(MY) -> M/1, To Workspace4/1
  Muq/1 -> My/6(Muq)
  Saturation3/1 -> Mqq2/1
  Saturation2/1 -> Mwq/1
  MATLAB Function2/1(y) -> Product5/1
  Selector8/1 -> Product5/2
  Product5/1 -> Saturation2/1
  Product4/1 -> Muq/1
  Mwq/1 -> My/5(Mwq)
  Mqq2/1 -> My/4(Mqq)
  dX/1 -> Mdxi/1(dX)
  dmass/1 -> My/12(dmass)
  dLCG/1 -> My/11(dLCG)
  Umag/1 -> My/9(Umag)
  Alpha/1 -> M'uvw/1
  Selector4/1 -> Product4/2, Saturation3/1, MATLAB Function2/1(u)
  UeX/1 -> My/10(UeX)
  M'prop/1 -> My/7(Mprop)
  Ba/1 -> My/3(Ba)
  Selector10/1 -> M'prop/1, M'uvw/2, Product4/1, Muq/2
  Bx/1 -> Selector2/1, My/1(Bx)
  Bv/1 -> My/2(Bv), Selector8/1, Selector4/1, Selector10/1

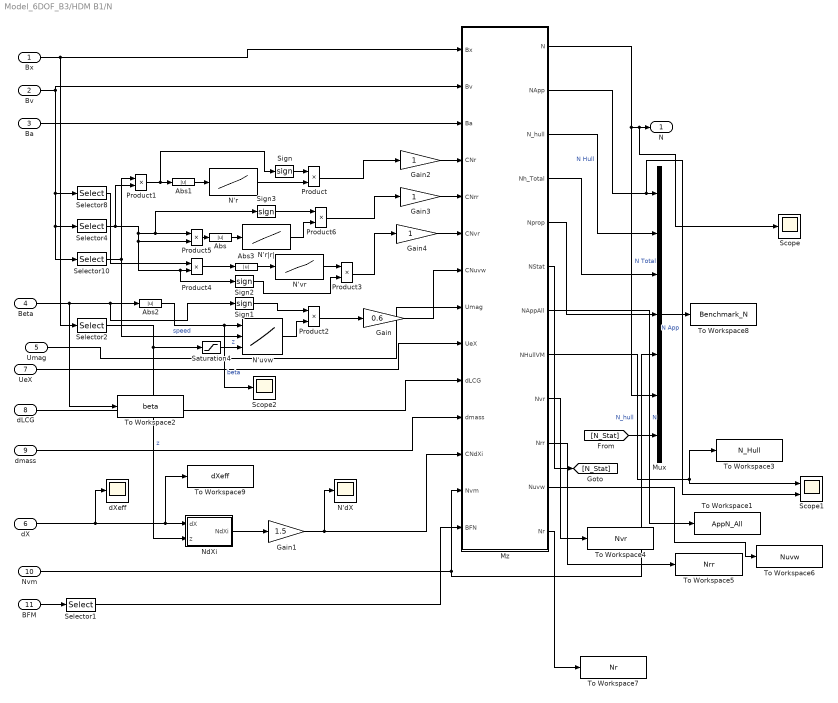
== system Model_6DOF_B3/HDM B1/N ==
  Bx : Inport
  Bv : Inport  Port=2
  Ba : Inport  Port=3
  Beta : Inport  Port=4
  Umag : Inport  Port=5
  dX : Inport  Port=6
  UeX : Inport  Port=7
  dLCG : Inport  Port=8
  dmass : Inport  Port=9
  Nvm : Inport  Port=10
  BFM : Inport  Port=11
  Abs{,1..3} (4 alike) : Abs
  Gain : Gain  Gain=0.6
  Gain1 : Gain  Gain=1.5
  Gain2 : Gain
  Gain3 : Gain
  Gain4 : Gain
  Mux : Mux  Inputs=7
  Mz : MATLAB Function  TreatAsAtomicUnit=on
  N'dX : Scope
  N'r : Lookup_n-D  NumberOfTableDimensions=1  BreakpointsForDimension1=|  Table=|  InternalRulePriority=Speed  RndMeth=Simplest  InputSameDT=on
      BreakpointsForDimension1=|
      | [0.03999989
      | 0.079999993
      | 0.11999963
      | 0.15999956]
      Table=|
      | [-4.0344E-04
      | -8.1402E-04
      | -1.2116E-03
      | -1.6125E-03]
  N'r|r| : Lookup_n-D  NumberOfTableDimensions=1  BreakpointsForDimension1=|  Table=|  InternalRulePriority=Speed  RndMeth=Simplest  InputSameDT=on
      BreakpointsForDimension1=|
      | [0.0001
      | 0.0003
      | 0.0006
      | 0.0009
      | 0.0012
      | 0.0015
      | ]
      Table=|
      | [1.93E-01
      | 6.44E-02
      | 3.19E-02
      | 2.11E-02
      | 1.64E-02
      | 1.34E-02
      | ]
  N'uvw : Lookup_n-D  NumberOfTableDimensions=3  BreakpointsForDimension1=|  BreakpointsForDimension2=|  BreakpointsForDimension3=|  Table=|  InternalRulePriority=Speed  RndMeth=Simplest  InputSameDT=on
      BreakpointsForDimension1=|
      | [0
      | 4
      | 8
      | 12]
      BreakpointsForDimension2=|
      | [-5.1444E+00
      | -3.0866E+00
      | -1.5433E+00
      | ]
      Table=|
      | reshape([0.0000000E+00
      | 1.1975814E-03
      | 2.7970643E-03
      | 4.1308534E-03
      | 0.0000000E+00
      | 1.2111628E-03
      | 2.9207146E-03
      | 4.1207837E-03
      | 0.0000000E+00
      | 1.4959851E-03
      | 2.9486406E-03
      | 4.1213058E-03
      | 0.0000000E+00
      | 1.4879743E-03
      | 2.9975710E-03
      | 4.2577903E-03
      | 0.0000000E+00
      | 1.4933232E-03
      | 3.0017417E-03
      | 4.2334501E-03
      | 0.0000000E+00
      | 1.5365285E-03
      | 3.0446384E-03
      | 4.4091424E-03
      | 0.0000000E+00
      | 1.5329300E-03
      | 3.0664177E-03
      | 4.3937198E-03
      | 0.0000000E+00
      | 1.5274021E-03
      | 3.0742094E-03
      | 4.3066710E-03
      | 0.0000000E+00
      | 1.5692494E-03
      | 3.1052278E-03
      | 4.3211963E-03
      | 0.0000000E+00
      | 1.5996020E-03
      | 3.2227652E-03
      | 4.5425478E-03
      | 0.0000000E+00
      | 1.5650123E-03
      | 3.1236229E-03
      | 4.4022471E-03
      | 0.0000000E+00
      | 1.6041810E-03
      | 3.1241151E-03
      | 4.4103656E-03],[4,3,4])
      BreakpointsForDimension3=|
      | [-35.0624 -18.3724 -15.3724 -13.8724
      | ]
      settings: InputPortMap=u0,u1,u2
  N'vr : Lookup_n-D  NumberOfTableDimensions=1  BreakpointsForDimension1=|  Table=|  InternalRulePriority=Speed  RndMeth=Simplest  InputSameDT=on
      BreakpointsForDimension1=|
      | [0
      | 0.051444
      | 0.102888
      | 0.205776
      | 0.411552]
      Table=|
      | [0.0000E+00
      | -1.9921E-03
      | -9.2025E-03
      | -3.2154E-02
      | -1.3255E-01]
  NdXi : Subsystem
  Product{,1..6} (7 alike) : Product
  Saturation4 : Saturate  UpperLimit=-13.8724  LowerLimit=-35.0624
  Scope : Scope
  Scope1 : Scope  NumInputPorts=2
  Scope2 : Scope
  Selector1 : Selector  InputPortWidth=6  IndexOptions=Index vector (dialog)  Indices=6  OutputSizes=1
  Selector10 : Selector  InputPortWidth=6  IndexOptions=Index vector (dialog)  Indices=1  OutputSizes=1
  Selector2 : Selector  InputPortWidth=6  IndexOptions=Index vector (dialog)  Indices=3  OutputSizes=1
  Selector4 : Selector  InputPortWidth=6  IndexOptions=Index vector (dialog)  Indices=6  OutputSizes=1
  Selector8 : Selector  InputPortWidth=6  IndexOptions=Index vector (dialog)  Indices=2  OutputSizes=1
  Sign{,1..3} (4 alike) : Signum
  To Workspace1 : ToWorkspace  VariableName=AppN_All  SaveFormat=Timeseries  SampleTime=-1
  To Workspace2 : ToWorkspace  VariableName=beta  SaveFormat=Timeseries  SampleTime=-1
  To Workspace3 : ToWorkspace  VariableName=N_Hull  SaveFormat=Timeseries  SampleTime=-1
  To Workspace4 : ToWorkspace  VariableName=Nvr  SaveFormat=Timeseries  SampleTime=-1
  To Workspace5 : ToWorkspace  VariableName=Nrr  SaveFormat=Timeseries  SampleTime=-1
  To Workspace6 : ToWorkspace  VariableName=Nuvw  SaveFormat=Timeseries  SampleTime=-1
  To Workspace7 : ToWorkspace  VariableName=Nr  SaveFormat=Timeseries  SampleTime=-1
  To Workspace8 : ToWorkspace  VariableName=Benchmark_N  SaveFormat=Timeseries  SampleTime=-1
  To Workspace9 : ToWorkspace  VariableName=dXeff  SaveFormat=Timeseries  SampleTime=-1
  dXeff : Scope
  N : Outport
  wires:
  Mz/12(Nr) -> To Workspace7/1
  Abs/1 -> N'r|r|/1
  Mz/11(Nuvw) -> To Workspace6/1
  Mz/10(Nrr) -> To Workspace5/1
  Mz/9(Nvr) -> To Workspace4/1
  Sign3/1 -> Product6/1
  Product6/1 -> Gain3/1
  Sign2/1 -> Product3/2
  N'vr/1 -> Product3/1
  Abs3/1 -> N'vr/1
  Mz/8(NHullVM) -> Scope1/1, To Workspace3/1  "N_hull"
  Saturation4/1 -> N'uvw/3  "z"
  Gain4/1 -> Mz/6(CNvr)
  Gain3/1 -> Mz/5(CNrr)
  Gain2/1 -> Mz/4(CNr)
  Mz/6(NStat) -> [N_Stat]
  [N_Stat] -> Mux/7
  Selector1/1 -> Mz/14(BFN)
  BFM/1 -> Selector1/1
  Mz/7(NAppAll) -> To Workspace1/1  "N"
  Mux/1 -> To Workspace8/1
  Mz/5(Nprop) -> Mux/4
  Mz/4(Nh_Total) -> Mux/3
  Mz/3(N_hull) -> Mux/2  "N Hull"
  Mz/2(NApp) -> Mux/1, Scope1/2  "N App"
  Nvm/1 -> Mz/13(Nvm), Mux/5
  Gain1/1 -> Mz/12(CNdXi), N'dX/1
  NdXi/1(NdXi) -> Gain1/1
  Gain/1 -> Mz/7(CNuvw)
  Product2/1 -> Gain/1
  Sign1/1 -> Product2/1
  Abs2/1 -> N'uvw/1, Scope2/1  "beta"
  Product/1 -> Gain2/1
  Sign/1 -> Product/1
  Abs1/1 -> N'r/1
  Product1/1 -> Abs1/1, Sign/1
  N'uvw/1 -> Product2/2
  Selector2/1 -> Saturation4/1, NdXi/2(z)  "z"
  Mz/1(N) -> Mux/6, N/1, Scope/1  "N Total"
  Product3/1 -> Gain4/1
  Product5/1 -> Abs/1
  Selector4/1 -> Sign3/1, Product5/1, Product5/2, Product4/2, Sign2/1, Product1/2
  Selector8/1 -> Product4/1
  Product4/1 -> Abs3/1
  N'r|r|/1 -> Product6/2
  N'r/1 -> Product/2
  dX/1 -> NdXi/1(dX), To Workspace9/1, dXeff/1
  dmass/1 -> Mz/11(dmass)
  dLCG/1 -> Mz/10(dLCG)
  Umag/1 -> Mz/8(Umag)
  Beta/1 -> To Workspace2/1, Abs2/1, Sign1/1
  UeX/1 -> Mz/9(UeX)
  Ba/1 -> Mz/3(Ba)
  Selector10/1 -> Product1/1, N'uvw/2  "speed"
  Bx/1 -> Selector2/1, Mz/1(Bx)
  Bv/1 -> Mz/2(Bv), Selector8/1, Selector4/1, Selector10/1

== system Model_6DOF_B3/HDM B1/Wave, Virtual Mass and Hydrostatic ==
  Bx_earth : Inport
  Bv_ship : Inport  Port=2
  SeaState : Inport  Port=3
  dLCG : Inport  Port=4
  Ba_ship : Inport  Port=5
  Add : Sum  Inputs=+-
  Add1 : Sum  Inputs=+-
  CG : Constant  Value=[32.3114 0 0]
  CGi : Constant  Value=|
      | [5.0784E+00	0.0000E+00	8.0728E-03;
      | 1.1013E+01	0.0000E+00	2.5384E-01;
      | 1.7302E+01	0.0000E+00	3.0728E-01;
      | 2.5741E+01	0.0000E+00	4.1417E-01;
      | 3.4688E+01	0.0000E+00	4.1585E-01;
      | 4.2324E+01	0.0000E+00	3.2444E-01;
      | 4.9992E+01	0.0000E+00	3.3454E-01;
      | 5.7427E+01	0.0000E+00	1.7420E-02;
      | 6.3078E+01	0.0000E+00	1.8824E-02;
      | 6.6703E+01	0.0000E+00	1.1340E-02;
      | 2.5141E+01	0.0000E+00	8.6491E+00;
      | 2.1732E+01	0.0000E+00	9.7273E+00;
      | 6.3166E+01	0.0000E+00	-4.0823E-17;
      | 2.2043E+01	0.0000E+00	9.7261E+00;
      | 6.3451E+01	0.0000E+00	-6.2238E-17;
      | ]
  Cvm*dm Plateau : Constant  Value=|
      | [8.4658E+04	1.7229E+05	1.6487E+05
      | 2.3551E+04	4.3394E+05	3.6176E+05
      | 1.1585E+03	5.9767E+05	4.2996E+05
      | 1.4123E+02	1.1354E+06	6.5606E+05
      | 9.1503E+01	6.9712E+05	5.1688E+05
      | 9.6110E+01	6.7201E+05	5.1905E+05
      | 1.2163E+04	5.7818E+05	4.7547E+05
      | 3.7219E+04	3.4697E+05	3.3508E+05
      | 1.9318E+04	7.7284E+04	7.6560E+04
      | 1.5368E+04	2.6375E+04	2.6268E+04
      | 1.8312E+04	4.5870E+05	5.1108E+04
      | 3.1859E+02	1.2645E+04	3.4886E+02
      | 3.0285E+03	4.4945E+04	4.4489E+04
      | 7.9160E+02	8.8963E+02	1.3306E+04
      | 1.2115E+03	3.9547E+04	3.9205E+04
      | ]
  Demux : Demux  Outputs=3
  Demux1 : Demux  Outputs=3
  Derivative : Derivative
  Derivative1 : Derivative
  Gain : Gain
  MATLAB Function : MATLAB Function  TreatAsAtomicUnit=on
  MATLAB Function1 : MATLAB Function  TreatAsAtomicUnit=on
  Manual Switch : ManualSwitch
  Manual Switch1 : ManualSwitch  CurrentSetting=0
  Wave Particle Motions : Subsystem
  Xvm : Outport
  Yvm : Outport  Port=2
  Zvm : Outport  Port=3
  Kvm : Outport  Port=4
  Mvm : Outport  Port=5
  Nvm : Outport  Port=6
  z_eff : Outport  Port=7
  uwsXi : Outport  Port=8
  uwsCG : Outport  Port=9
  B_FM : Outport  Port=10
  wires:
  Gain/1 -> MATLAB Function/1(cvm)
  Wave Particle Motions/9(B_FM) -> B_FM/1
  Manual Switch1/1 -> MATLAB Function/2(Awrs)
  Add1/1 -> Manual Switch1/1  "d/dt(aw)-d/dt(ar)"
  Derivative1/1 -> Manual Switch1/2  "d/dt(aw-ar)"
  Add/1 -> Derivative1/1
  Wave Particle Motions/8(urs) -> Add/2
  Wave Particle Motions/7(uws) -> Add/1
  MATLAB Function1/1(Fvm) -> Manual Switch/2
  Manual Switch/1 -> Demux/1
  Ba_ship/1 -> MATLAB Function1/2(asCG)
  Derivative/1 -> MATLAB Function1/1(awsCG)
  Cvm*dm Plateau/1 -> Gain/1
  Wave Particle Motions/6(uwsCG) -> uwsCG/1, Derivative/1
  Wave Particle Motions/5(uwXis) -> uwsXi/1
  Demux1/3 -> Nvm/1
  Demux1/1 -> Kvm/1
  Demux1/2 -> Mvm/1
  Demux/3 -> Zvm/1
  Demux/2 -> Yvm/1
  Demux/1 -> Xvm/1
  MATLAB Function/8(Mvm) -> Demux1/1  "Mvm"
  MATLAB Function/7(Fvm) -> Manual Switch/1  "Fvm"
  Bv_ship/1 -> Wave Particle Motions/1(U_ship)
  dLCG/1 -> Wave Particle Motions/6(dLCG)
  SeaState/1 -> Wave Particle Motions/5(SeaState)
  Wave Particle Motions/3(Rs) -> MATLAB Function/3(Rs)
  CG/1 -> Wave Particle Motions/4(CG)
  CGi/1 -> Wave Particle Motions/3(CGi)
  Wave Particle Motions/1(aws) -> Add1/1
  Wave Particle Motions/2(ars) -> Add1/2
  Bx_earth/1 -> Wave Particle Motions/2(X_earth)
  Wave Particle Motions/4(zeff) -> z_eff/1
